simulink model "SF_Integral_Action_Simulation"  (R2021b)
settings: Solver=VariableStepAuto  StartTime=0.0  StopTime=20  RelTol=1e-3
undefined symbols (not defined in the file): Ad, Bd, Cd, ki, Kp, L, Ts
libraries: cstblocks x1
settings Model: Creator=UTENTE  LastModifiedBy=UTENTE

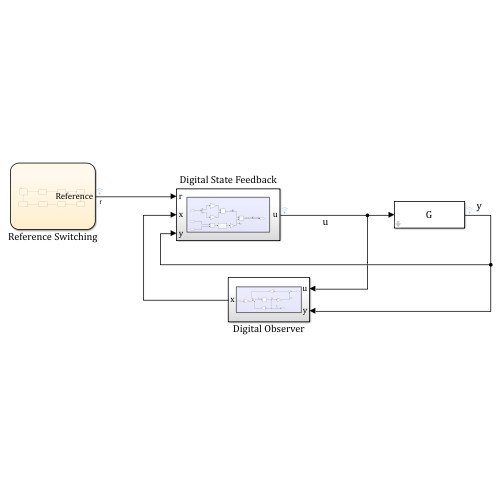
[thumbnail: Simulink's stored preview of the top-level diagram]
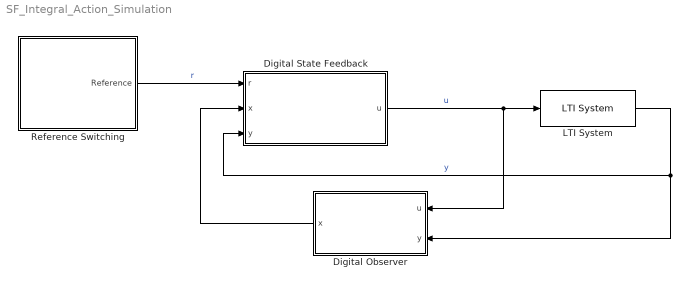
== system SF_Integral_Action_Simulation ==
  Digital Observer : Subsystem
  Digital State Feedback : Subsystem
  LTI System : cstblocks/LTI System  sys=G  IC=[]
  Reference Switching : Stateflow chart  TreatAsAtomicUnit=on
  wires:
  Digital State Feedback/1(u) -> Digital Observer/1(u), LTI System/1  "u"
  LTI System/1 -> Digital State Feedback/3(y), Digital Observer/2(y)  "y"
  Digital Observer/1(x) -> Digital State Feedback/2(x)
  Reference Switching/1(Reference) -> Digital State Feedback/1(r)  "r"

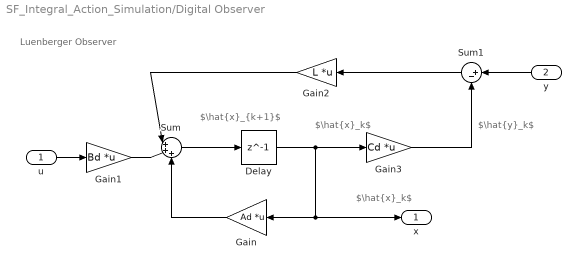
== system SF_Integral_Action_Simulation/Digital Observer ==
  note: $\hat{x}_{k+1}$
  note: Luenberger Observer
  note: $\hat{x}_k$
  note: $\hat{y}_k$
  note: $\hat{x}_k$
  u : Inport
  y : Inport  Port=2
  Delay : Delay  DelayLength=1  SampleTime=Ts
  Gain : Gain  Gain=Ad  Multiplication=Matrix(K*u)
  Gain1 : Gain  Gain=Bd  Multiplication=Matrix(K*u)
  Gain2 : Gain  Gain=L  Multiplication=Matrix(K*u)
  Gain3 : Gain  Gain=Cd  Multiplication=Matrix(K*u)
  Sum : Sum  Inputs=|+++
  Sum1 : Sum  Inputs=|+-
  x : Outport
  wires:
  u/1 -> Gain1/1
  Gain3/1 -> Sum1/2
  Delay/1 -> x/1, Gain/1, Gain3/1
  Gain1/1 -> Sum/2
  Gain2/1 -> Sum/1
  Sum/1 -> Delay/1
  Gain/1 -> Sum/3
  Sum1/1 -> Gain2/1
  y/1 -> Sum1/1

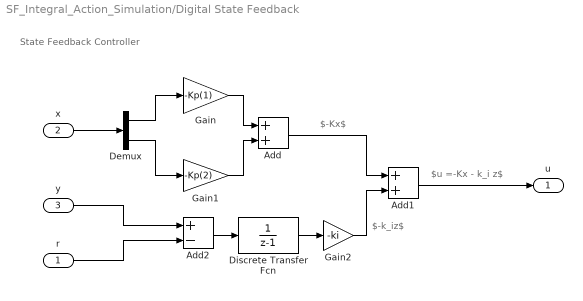
== system SF_Integral_Action_Simulation/Digital State Feedback ==
  note: $u =-Kx - k_i z$
  note: $-k_iz$
  note: $-Kx$
  note: State Feedback Controller
  r : Inport
  x : Inport  Port=2
  y : Inport  Port=3
  Add : Sum
  Add1 : Sum
  Add2 : Sum  Inputs=+-
  Demux : Demux  Outputs=2
  Discrete Transfer Fcn : DiscreteTransferFcn  Denominator=[1 -1]  SampleTime=Ts
  Gain : Gain  Gain=-Kp(1)
  Gain1 : Gain  Gain=-Kp(2)
  Gain2 : Gain  Gain=-ki
  u : Outport
  wires:
  Gain/1 -> Add/1
  y/1 -> Add2/1
  Discrete Transfer Fcn/1 -> Gain2/1
  Gain2/1 -> Add1/2
  Add2/1 -> Discrete Transfer Fcn/1
  x/1 -> Demux/1
  r/1 -> Add2/2
  Demux/2 -> Gain1/1
  Gain1/1 -> Add/2
  Add1/1 -> u/1
  Add/1 -> Add1/1
  Demux/1 -> Gain/1

== stateflow chart SF_Integral_Action_Simulation/Reference Switching ==
  state S1
    Reference=0;
  state S2
    Reference=80;
  state S3
    Reference=125;
  state s4
    Reference=150;
  state s7
    Reference=-125;
  state s8
    Reference=-150;
  state s6
    Reference=-80
  state s5
    Reference=0
  (default) -> S1
  S1 -> S2 : after(2,sec)
  S2 -> S3 : after(2,sec)
  S3 -> s4 : after(2,sec)
  s4 -> s5 : after(2,sec)
  s8 -> S1 : after(2,sec)
  s7 -> s8 : after(2,sec)
  s6 -> s7 : after(2,sec)
  s5 -> s6 : after(2,sec)
  data: Reference output
